simulink model "DC-motor-analogue-control"  (R2017a)
settings: Solver=VariableStepAuto  StartTime=0.0  StopTime=50  RelTol=1e-3
libraries: simulink x1
settings Model: Creator=Michy  LastModifiedBy=Michy

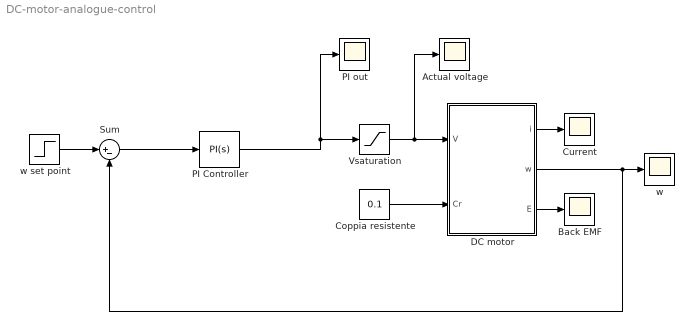
== system DC-motor-analogue-control ==
  Actual voltage : Scope
  Back EMF : Scope
  Coppia resistente : Constant  Value=0.1
  Current : Scope
  DC motor : Subsystem  mask{L=0.0028, R=5.5, k=1, phi=0.5, J=0.5}
      mask prompts: L "L [H]"; R "R [Ohm]"; phi "phi [Wb]"; J "J [kg m^2]"
  PI Controller : simulink/Continuous/PID Controller  Controller=PI  TimeDomain=Continuous-time  SampleTime=-1  IntegratorMethod=Forward Euler  FilterMethod=Forward Euler  Form=Parallel  UseFilter=on  ControllerParametersSource=internal  P=5.68484714598179  I=1.72471430989899  D=0  N=100  InitialConditionSource=internal  InitialConditionForIntegrator=0  InitialConditionForFilter=0  ExternalReset=none  LimitOutput=off  UpperSaturationLimit=inf  LowerSaturationLimit=-inf  LinearizeAsGain=on  AntiWindupMode=none  Kb=1  TrackingMode=off  Kt=1  PParamMin=[]  PParamMax=[]  IParamMin=[]  IParamMax=[]  DParamMin=[]  DParamMax=[]  NParamMin=[]  NParamMax=[]  KbParamMin=[]  KbParamMax=[]  KtParamMin=[]  KtParamMax=[]  POutMin=[]  POutMax=[]  IOutMin=[]  IOutMax=[]  DOutMin=[]  DOutMax=[]  NOutMin=[]  NOutMax=[]  KbOutMin=[]  KbOutMax=[]  KtOutMin=[]  KtOutMax=[]  IntegratorOutMin=[]  IntegratorOutMax=[]  FilterOutMin=[]  FilterOutMax=[]  SumOutMin=[]  SumOutMax=[]  SumI1OutMin=[]  SumI1OutMax=[]  SumI2OutMin=[]  SumI2OutMax=[]  SumI3OutMin=[]  SumI3OutMax=[]  SumDOutMin=[]  SumDOutMax=[]  SaturationOutMin=[]  SaturationOutMax=[]  IntegratorContinuousStateAttributes=''  IntegratorStateMustResolveToSignalObject=off  IntegratorRTWStateStorageClass=Auto  FilterContinuousStateAttributes=''  FilterStateMustResolveToSignalObject=off  FilterRTWStateStorageClass=Auto  DifferentiatorICPrevScaledInput=0  DifferentiatorOutMin=[]  DifferentiatorOutMax=[]  InitialConditionSetting=State (most efficient)
  PI out : Scope
  Sum : Sum  Inputs=|+-
  Vsaturation : Saturate  UpperLimit=24  LowerLimit=0
  w : Scope
  w set point : Step  Time=20  Before=10  After=5  SampleTime=0
  wires:
  Coppia resistente/1 -> DC motor/2(Cr)
  DC motor/2(w) -> Sum/2, w/1
  DC motor/1(i) -> Current/1
  DC motor/3(E) -> Back EMF/1
  w set point/1 -> Sum/1
  Vsaturation/1 -> DC motor/1(V), Actual voltage/1
  PI Controller/1 -> PI out/1, Vsaturation/1
  Sum/1 -> PI Controller/1

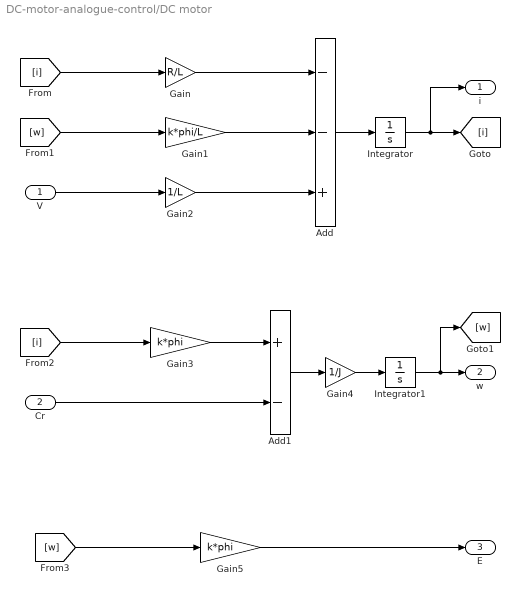
== system DC-motor-analogue-control/DC motor ==
  V : Inport
  Cr : Inport  Port=2
  Add : Sum  Inputs=--+
  Add1 : Sum  Inputs=+-
  Gain : Gain  Gain=R/L
  Gain1 : Gain  Gain=k*phi/L
  Gain2 : Gain  Gain=1/L
  Gain3 : Gain  Gain=k*phi
  Gain4 : Gain  Gain=1/J
  Gain5 : Gain  Gain=k*phi
  Integrator : Integrator
  Integrator1 : Integrator
  i : Outport
  w : Outport  Port=2
  E : Outport  Port=3
  wires:
  [i] -> Gain/1
  [w] -> Gain1/1
  V/1 -> Gain2/1
  Gain/1 -> Add/1
  Gain1/1 -> Add/2
  Gain2/1 -> Add/3
  Add/1 -> Integrator/1
  Integrator/1 -> i/1, [i]
  [i] -> Gain3/1
  Gain3/1 -> Add1/1
  Cr/1 -> Add1/2
  Add1/1 -> Gain4/1
  Gain4/1 -> Integrator1/1
  Integrator1/1 -> [w], w/1
  [w] -> Gain5/1
  Gain5/1 -> E/1
